simulink model "Simulatore"  (R2023a)
settings: Solver=VariableStepAuto  StartTime=0.0  StopTime=35  RelTol=1e-3
values from neighbouring files (symbols this model uses):
  BC = [bc11 bc12; bc21 bc22]    [Parametri.m]
  BV = [bv11 bv12; bv21 bv22]    [Parametri.m]
  G1 = (m1*l1+m2*a1)*g    (= 13.72)    [Parametri.m]
  G2 = m2*l2*g    (= 3.136)    [Parametri.m]
  GG1 = (mm1*l1+mm2*a1)*g    (= 12.789)    [Parametri.m]
  GG2 = mm2*l2*g    (= 2.8616)    [Parametri.m]
  H = -m2*a1*l2    (= -0.32)    [Parametri.m]
  HH = -mm2*a1*l2    (= -0.292)    [Parametri.m]
  L = [a1;a2]    [Parametri.m]
  P1 = [0.5; 0.3]    [Parametri.m]
  P2 = [1.5; 0.3]    [Parametri.m]
  q10 = Q(1)    [Parametri.m]
  q20 = Q(2)    [Parametri.m]
  T = [10;30]    [Parametri.m]
(part 2 of 2)

== matlab function Simulatore/Dinamica4/gravity ==
  data: G1 input; G output; G2 input; q1 input; q2 input
function G = fcn(G1, G2, q1, q2)
c1=cos(q1);
c12=cos(q1+q2);

G = [G1*c1+G2*c12; G2*c12];

== matlab function Simulatore/Dinamica4/inversa1 ==
  data: HH input; u1 output; B input; G input; T1 input; u2 output; T2 input
function [u1,u2] = fcn(HH,B,G,T1,T2)

y =inv(B)*[[T1;T2]-HH-G];
u1=y(1);
u2=y(2);

== matlab function Simulatore/Generatore di riferimenti4/MATLAB Function ==
  data: P1 input; P output; P2 input; T input; t input
function P = genera_riferimenti(P1,P2,T,t)

t1 = T(1);
t2 = T(2);
P1x = P1(1);
P1y = P1(2);
P2x = P2(1);
P2y = P2(2);

P=[0;0];

cx = 1;
cy = 0.3;
r = 0.5;


if ( t>t2 )
    P(1) = P1x;
    P(2) = P1y;
    
end

if ( t1>=t )
    sigma_r = (t-0)/(t1-0);
    lambda_r = -20*sigma_r^7+70*sigma_r^6-84*sigma_r^5+35*sigma_r^4;
    P(1) = P1x + lambda_r*(P2x - P1x);
    P(2) = P1y + lambda_r*(P2y - P1y);

end

if ( t>t1 && t<=t2)
    sigma_c = (t-t1)/(t2-t1);
    lambda_c = -20*sigma_c^7+70*sigma_c^6-84*sigma_c^5+35*sigma_c^4;
    theta0 = 0;
    theta1 = pi;
    theta = theta0 + lambda_c*(theta1-theta0);
    P(1) = cx + r*cos(theta);
    P(2) = cy + r*sin(theta);
end

end

== matlab function Simulatore/Generatore di riferimenti4/MATLAB Function1 ==
  data: P input; q1 output; q2 output; L input
function [q1, q2] = cinematica_inversa(P,L)
L1=L(1);
L2=L(2);
x=P(1);
y=P(2);

c2=(x^2+y^2-L1^2-L2^2)/2/L1/L2;

s2=sqrt(1-c2^2);
if c2==-1
    s2=1;
end
q2=atan2(s2,c2);
A=[L1+L2*c2 -L2*s2; 
    L2*s2 (L1+L2*c2)];
Q1=inv(A)*P;
c1=Q1(1);
s1=Q1(2);
q1=atan2(s1,c1);

end

== matlab function Simulatore/MATLAB Function4 ==
  data: L input; x output; q1 input; y output; q2 input
function [x,y] = cinematica_diretta(L, q1,q2)
L1=L(1);
L2=L(2);
x=L1*cos(q1)+L2*cos(q1+q2);
y=L1*sin(q1)+L2*sin(q1+q2);

== matlab function Simulatore/Controllore con compensazione perfetta delle forze apparenti/MATLAB Function ==
  data: H input; q2 input; H1 output; qd1 input; qd2 input; H2 output
function [H1, H2] = forze_apparenti(H, q2, qd1, qd2)
uu1=H*sin(q2);
h =uu1*[(2*qd1*qd2+qd2^2); -qd1^2];
H1 = h(1);
H2 = h(2);

== matlab function Simulatore/Controllore con compensazione perfetta delle forze apparenti/MATLAB Function1 ==
  data: G1 input; GG1 output; G2 input; q1 input; q2 input; GG2 output
function [GG1, GG2] = gravita(G1, G2, q1, q2)
c1 = cos(q1);
c12 = cos(q1+q2);
G = [G1*c1+G2*c12; G2*c12];

GG1 = G(1);
GG2 = G(2);

== matlab function Simulatore/Dinamica5/B1 ==
  data: qq2 input; B output; BC input; BV input
function B = fcn(qq2,BC,BV)
B=BC+cos(qq2)*BV;

== matlab function Simulatore/Generatore di riferimenti/MATLAB Function ==
  data: P1 input; P output; P2 input; T input; t input
function P = genera_riferimenti(P1,P2,T,t)

t1 = T(1);
t2 = T(2);
P1x = P1(1);
P1y = P1(2);
P2x = P2(1);
P2y = P2(2);

P=[0;0];
                
cx = 1;
cy = 0.3;
r = 0.5;


if ( t>t2 )
    P(1) = P1x;
    P(2) = P1y;
    
end

if ( t1>=t )
    sigma_r = (t-0)/(t1-0);
    lambda_r = -20*sigma_r^7+70*sigma_r^6-84*sigma_r^5+35*sigma_r^4;
    P(1) = P1x + lambda_r*(P2x - P1x);
    P(2) = P1y + lambda_r*(P2y - P1y);

end

if ( t>t1 && t<=t2)
    sigma_c = (t-t1)/(t2-t1);
    lambda_c = -20*sigma_c^7+70*sigma_c^6-84*sigma_c^5+35*sigma_c^4;
    theta0 = 0;
    theta1 = pi;
    theta = theta0 + lambda_c*(theta1-theta0);
    P(1) = cx + r*cos(theta);
    P(2) = cy + r*sin(theta);
end

end

== matlab function Simulatore/Dinamica5/HH1 ==
  data: H input; qq2 input; HH output; qd1 input; qd2 input
function HH = fcn(H,qq2,qd1,qd2)
Hs2=H*sin(qq2);
HH =Hs2*[(2*qd1*qd2+qd2^2); -qd1^2];

== matlab function Simulatore/Dinamica5/gravity ==
  data: G1 input; G output; G2 input; q1 input; q2 input
function G = fcn(G1, G2, q1, q2)
c1=cos(q1);
c12=cos(q1+q2);

G = [G1*c1+G2*c12; G2*c12];

== matlab function Simulatore/Dinamica5/inversa1 ==
  data: HH input; u1 output; B input; G input; T1 input; u2 output; T2 input
function [u1,u2] = fcn(HH,B,G,T1,T2)

y =inv(B)*[[T1;T2]-HH-G];
u1=y(1);
u2=y(2);

== matlab function Simulatore/Generatore di riferimenti5/MATLAB Function ==
  data: P1 input; P output; P2 input; T input; t input
function P = genera_riferimenti(P1,P2,T,t)

t1 = T(1);
t2 = T(2);
P1x = P1(1);
P1y = P1(2);
P2x = P2(1);
P2y = P2(2);

P=[0;0];

cx = 1;
cy = 0.3;
r = 0.5;


if ( t>t2 )
    P(1) = P1x;
    P(2) = P1y;
    
end

if ( t1>=t )
    sigma_r = (t-0)/(t1-0);
    lambda_r = -20*sigma_r^7+70*sigma_r^6-84*sigma_r^5+35*sigma_r^4;
    P(1) = P1x + lambda_r*(P2x - P1x);
    P(2) = P1y + lambda_r*(P2y - P1y);

end

if ( t>t1 && t<=t2)
    sigma_c = (t-t1)/(t2-t1);
    lambda_c = -20*sigma_c^7+70*sigma_c^6-84*sigma_c^5+35*sigma_c^4;
    theta0 = 0;
    theta1 = pi;
    theta = theta0 + lambda_c*(theta1-theta0);
    P(1) = cx + r*cos(theta);
    P(2) = cy + r*sin(theta);
end

end

== matlab function Simulatore/Generatore di riferimenti5/MATLAB Function1 ==
  data: P input; q1 output; q2 output; L input
function [q1, q2] = cinematica_inversa(P,L)
L1=L(1);
L2=L(2);
x=P(1);
y=P(2);

c2=(x^2+y^2-L1^2-L2^2)/2/L1/L2;

s2=sqrt(1-c2^2);
if c2==-1
    s2=1;
end
q2=atan2(s2,c2);
A=[L1+L2*c2 -L2*s2; 
    L2*s2 (L1+L2*c2)];
Q1=inv(A)*P;
c1=Q1(1);
s1=Q1(2);
q1=atan2(s1,c1);

end

== matlab function Simulatore/MATLAB Function5 ==
  data: L input; x output; q1 input; y output; q2 input
function [x,y] = cinematica_diretta(L, q1,q2)
L1=L(1);
L2=L(2);
x=L1*cos(q1)+L2*cos(q1+q2);
y=L1*sin(q1)+L2*sin(q1+q2);

== matlab function Simulatore/Dinamica/B1 ==
  data: qq2 input; B output; BC input; BV input
function B = fcn(qq2,BC,BV)
B=BC+cos(qq2)*BV;

== matlab function Simulatore/Dinamica/HH1 ==
  data: H input; qq2 input; HH output; qd1 input; qd2 input
function HH = fcn(H,qq2,qd1,qd2)
Hs2 = H*sin(qq2);
HH = Hs2*[(2*qd1*qd2+qd2^2); -qd1^2];

== matlab function Simulatore/Dinamica1/inversa1 ==
  data: HH input; u1 output; B input; G input; T1 input; u2 output; T2 input
function [u1,u2] = fcn(HH,B,G,T1,T2)

y =inv(B)*[[T1;T2]-HH-G];
u1=y(1);
u2=y(2);

== matlab function Simulatore/Dinamica/inversa1 ==
  data: HH input; u1 output; B input; T1 input; u2 output; T2 input
function [u1,u2] = fcn(HH,B,T1,T2)

y =inv(B)*[[T1;T2]-HH];
u1=y(1);
u2=y(2);

== matlab function Simulatore/Generatore di riferimenti1/MATLAB Function ==
  data: P1 input; P output; P2 input; T input; t input
function P = genera_riferimenti(P1,P2,T,t)

t1 = T(1);
t2 = T(2);
P1x = P1(1);
P1y = P1(2);
P2x = P2(1);
P2y = P2(2);

P=[0;0];

cx = 1;
cy = 0.3;
r = 0.5;


if ( t>t2 )
    P(1) = P1x;
    P(2) = P1y;
    
end

if ( t1>=t )
    sigma_r = (t-0)/(t1-0);
    lambda_r = -20*sigma_r^7+70*sigma_r^6-84*sigma_r^5+35*sigma_r^4;
    P(1) = P1x + lambda_r*(P2x - P1x);
    P(2) = P1y + lambda_r*(P2y - P1y);

end

if ( t>t1 && t<=t2)
    sigma_c = (t-t1)/(t2-t1);
    lambda_c = -20*sigma_c^7+70*sigma_c^6-84*sigma_c^5+35*sigma_c^4;
    theta0 = 0;
    theta1 = pi;
    theta = theta0 + lambda_c*(theta1-theta0);
    P(1) = cx + r*cos(theta);
    P(2) = cy + r*sin(theta);
end

end
